simulink library "tpm"  (R2021b)
settings: Solver=VariableStepAuto  StartTime=0.0  StopTime=10.0  RelTol=1e-3
undefined symbols (not defined in the file or in its folder): ENUM_AN_LF, ENUM_AN_LR, ENUM_AN_RF, ENUM_AN_RR, ENUM_POWERSTA_OFF, ENUM_POWERSTA_OFFA, ENUM_POWERSTA_OFFC, ENUM_POWERSTA_ON, ENUM_POWERSTA_READY, ENUM_POWERSTA_STANDBY, ENUM_PWRSTASW_OFF, ENUM_PWRSTASW_OFFA, ENUM_PWRSTASW_OFFCHVCHRG, ENUM_PWRSTASW_STANDBY, ENUM_TPMSSNESORIDREGSTA_START, FALSE, KTPM_DataInVehSpdThreshold_kph, KTPM_Delay_raw8, KTPM_DiagLearn_flg, KTPM_TPMSModelVersion_raw, KTPM_TPMSModelVersionInit_raw, KTPM_WhlRotDir_enum_ovrdflg, KTPM_WhlRotDir_enum_ovrdval, TRUE, ZERO_FLOAT, ZERO_INT
libraries: simulink x58, $bdroot x27, hcu_lib x24
(part 8 of 9)

== stateflow chart tpm/TPM/TPMS/TPMS/Learn/AutoLocation/IDIdentify/Subsystem1/Chart ==
  state Sample [parallel]
    settings: executionOrder=1
    state DataNotEnough
    state Regisiter
      en:
      C=C+1;
      LFM=LF_PC;
      RFM=RF_PC;
      LRM=LR_PC;
      RRM=RR_PC;
    (default) -> DataNotEnough : {C=0;}
    Regisiter -> (junction 513) [order 2] : [GS]
    DataNotEnough -> Regisiter [order 2] : [!VINP_TPMSResButt_flg&&GS]
    (junction 513) -> (junction 514)
    (junction 514) -> Regisiter
    Regisiter -> DataNotEnough [order 1] : [VINP_TPMSResButt_flg]{C=0;}
    Regisiter -> (junction 528) [order 3] : [VPMM_PowerSta_enum!=ENUM_POWERSTA_ON&&...
        | VPMM_PowerSta_enum!=ENUM_POWERSTA_READY
        | ]
    (junction 528) -> (junction 532) : {C=0;}
    (junction 532) -> DataNotEnough
    DataNotEnough -> DataNotEnough [order 1] : [VINP_TPMSResButt_flg]{C=0;}
  data: VINP_TPMSResButt_flg input; VPMM_PowerSta_enum input; GS input; LR_PC input; LF_PC input; RR_PC input; RF_PC input; LFM output int16; LRM output int16; RRM output int16; RFM output int16; C output uint8; ENUM_POWERSTA_READY parameter; ENUM_POWERSTA_ON parameter

== matlab function tpm/TPM/TPMS/TPMS/Learn/AutoLocation/IDIdentify/Subsystem2/Enabled Subsystem1/MATLAB Function ==
  data: C input; S output; Min input; X2 input; X3 input; X4 input; Y2 output; Y3 output; Y4 output; X5 input; X6 input; X7 input; X8 input; X9 input; Y5 output; Y6 output; Y7 output; Y8 output; Y9 output
function [S,Y2,Y3,Y4,Y5,Y6,Y7,Y8,Y9]   = fcn(C,Min,X2,X3,X4,X5,X6,X7,X8,X9)
Y=int16([X2 X3 X4 X5 X6 X7 X8 X9 Min]);
if (C<9)
    S=300;
else
    B=sort(Y);
    D=zeros(1,length(B));
    for i=1:1:length(D)
        if (i~=length(D))
            D(i)=B(i+1)-B(i);
        else
            if (B(length(D))-B(1)>B(1)+96-B(length(D)))
                D(length(D))=B(1)+96-B(length(D));
            else
                D(length(D))=B(length(D))-B(1);
            end
        end
    end

    [K,I]=sort(D);
    S=sum(K(1:7));
end
Y2=Y(2);
Y3=Y(3);
Y4=Y(4);
Y5=Y(5);
Y6=Y(6);
Y7=Y(7);
Y8=Y(8);
Y9=Y(9);

== matlab function tpm/TPM/TPMS/TPMS/Learn/AutoLocation/IDIdentify/Subsystem2/Enabled Subsystem2/MATLAB Function ==
  data: C input; S output; Min input; X2 input; X3 input; X4 input; Y2 output; Y3 output; Y4 output; X5 input; X6 input; X7 input; X8 input; X9 input; Y5 output; Y6 output; Y7 output; Y8 output; Y9 output
function [S,Y2,Y3,Y4,Y5,Y6,Y7,Y8,Y9]   = fcn(C,Min,X2,X3,X4,X5,X6,X7,X8,X9)
Y=int16([X2 X3 X4 X5 X6 X7 X8 X9 Min]);
if (C<9)
    S=300;
else
    B=sort(Y);
    D=zeros(1,length(B));
    for i=1:1:length(D)
        if (i~=length(D))
            D(i)=B(i+1)-B(i);
        else
            if (B(length(D))-B(1)>B(1)+96-B(length(D)))
                D(length(D))=B(1)+96-B(length(D));
            else
                D(length(D))=B(length(D))-B(1);
            end
        end
    end

    [K,I]=sort(D);
    S=sum(K(1:7));
end
Y2=Y(2);
Y3=Y(3);
Y4=Y(4);
Y5=Y(5);
Y6=Y(6);
Y7=Y(7);
Y8=Y(8);
Y9=Y(9);

== matlab function tpm/TPM/TPMS/TPMS/Learn/AutoLocation/IDIdentify/Subsystem2/Enabled Subsystem3/MATLAB Function ==
  data: C input; S output; Min input; X2 input; X3 input; X4 input; Y2 output; Y3 output; Y4 output; X5 input; X6 input; X7 input; X8 input; X9 input; Y5 output; Y6 output; Y7 output; Y8 output; Y9 output
function [S,Y2,Y3,Y4,Y5,Y6,Y7,Y8,Y9]   = fcn(C,Min,X2,X3,X4,X5,X6,X7,X8,X9)
Y=int16([X2 X3 X4 X5 X6 X7 X8 X9 Min]);
if (C<9)
    S=300;
else
    B=sort(Y);
    D=zeros(1,length(B));
    for i=1:1:length(D)
        if (i~=length(D))
            D(i)=B(i+1)-B(i);
        else
            if (B(length(D))-B(1)>B(1)+96-B(length(D)))
                D(length(D))=B(1)+96-B(length(D));
            else
                D(length(D))=B(length(D))-B(1);
            end
        end
    end

    [K,I]=sort(D);
    S=sum(K(1:7));
end
Y2=Y(2);
Y3=Y(3);
Y4=Y(4);
Y5=Y(5);
Y6=Y(6);
Y7=Y(7);
Y8=Y(8);
Y9=Y(9);

== stateflow chart tpm/TPM/TPMS/TPMS/Learn/AutoLocation/Subsystem/Chart ==
  state writeSXID
    (default) -> (junction 6)
    writeSXID -> (junction 6)
    (junction 6) -> (junction 8) [order 1] : [VINP_TPMSResButt_flg]
    (junction 6) -> (junction 10) [order 2] : {
        | VTPM_FlashS1ID_raw=S1ID;
        | VTPM_FlashS2ID_raw=S2ID;
        | VTPM_FlashS3ID_raw=S3ID;
        | VTPM_FlashS4ID_raw=S4ID;
        | VTPM_FlashIDvalid_enum=1;
        | }
    (junction 8) -> (junction 12) : {
        | VTPM_FlashS1ID_raw=0;
        | VTPM_FlashS2ID_raw=0;
        | VTPM_FlashS3ID_raw=0;
        | VTPM_FlashS4ID_raw=0;
        | VTPM_FlashIDvalid_enum=0;
        | }
    (junction 12) -> (junction 10)
  data: S1ID input; S2ID input; S3ID input; S4ID input; VINP_TPMSResButt_flg input; VTPM_FlashS1ID_raw output uint32; VTPM_FlashS2ID_raw output uint32; VTPM_FlashS3ID_raw output uint32; VTPM_FlashS4ID_raw output uint32; VTPM_FlashIDvalid_enum output uint8

== matlab function tpm/TPM/TPMS/TPMS/Learn/AutoLocation/IDIdentify/Subsystem2/Enabled Subsystem5/MATLAB Function ==
  data: C input; S output; Min input; X2 input; X3 input; X4 input; Y2 output; Y3 output; Y4 output; X5 input; X6 input; X7 input; X8 input; X9 input; Y5 output; Y6 output; Y7 output; Y8 output; Y9 output
function [S,Y2,Y3,Y4,Y5,Y6,Y7,Y8,Y9]   = fcn(C,Min,X2,X3,X4,X5,X6,X7,X8,X9)
Y=int16([X2 X3 X4 X5 X6 X7 X8 X9 Min]);
if (C<9)
    S=300;
else
    B=sort(Y);
    D=zeros(1,length(B));
    for i=1:1:length(D)
        if (i~=length(D))
            D(i)=B(i+1)-B(i);
        else
            if (B(length(D))-B(1)>B(1)+96-B(length(D)))
                D(length(D))=B(1)+96-B(length(D));
            else
                D(length(D))=B(length(D))-B(1);
            end
        end
    end

    [K,I]=sort(D);
    S=sum(K(1:7));
end
Y2=Y(2);
Y3=Y(3);
Y4=Y(4);
Y5=Y(5);
Y6=Y(6);
Y7=Y(7);
Y8=Y(8);
Y9=Y(9);

== stateflow chart tpm/TPM/TPMS/TPMS/Learn/AutoLocation/IDIdentify/Subsystem3/Chart ==
  state Sample [parallel]
    settings: executionOrder=1
    state DataNotEnough
    state Regisiter
      en:
      C=C+1;
      LFM=LF_PC;
      RFM=RF_PC;
      LRM=LR_PC;
      RRM=RR_PC;
    (default) -> DataNotEnough : {C=0;}
    Regisiter -> (junction 513) [order 2] : [GS]
    DataNotEnough -> Regisiter [order 2] : [!VINP_TPMSResButt_flg&&GS]
    (junction 513) -> (junction 514)
    (junction 514) -> Regisiter
    Regisiter -> DataNotEnough [order 1] : [VINP_TPMSResButt_flg]{C=0;}
    Regisiter -> (junction 528) [order 3] : [VPMM_PowerSta_enum!=ENUM_POWERSTA_ON&&...
        | VPMM_PowerSta_enum!=ENUM_POWERSTA_READY
        | ]
    (junction 528) -> (junction 532) : {C=0;}
    (junction 532) -> DataNotEnough
    DataNotEnough -> DataNotEnough [order 1] : [VINP_TPMSResButt_flg]{C=0;}
  data: VINP_TPMSResButt_flg input; VPMM_PowerSta_enum input; GS input; LR_PC input; LF_PC input; RR_PC input; RF_PC input; LFM output int16; LRM output int16; RRM output int16; RFM output int16; C output uint8; ENUM_POWERSTA_READY parameter; ENUM_POWERSTA_ON parameter

== stateflow chart tpm/TPM/TPMS/TPMS/Learn/AutoLocation/IDIdentify/Subsystem3/Chart1 ==
  state GCal [parallel]
    settings: executionOrder=1
    state NoSignal
      en:G=false;
    state SignalIn
      en:G=true;
    (default) -> NoSignal
    NoSignal -> (junction 17) : [VINP_DATAin_flg]
    (junction 17) -> SignalIn [order 1] : [!Used]
    (junction 17) -> (junction 19) [order 2]
    (junction 19) -> NoSignal [order 2]
    (junction 19) -> SignalIn [order 1] : [VINP_IDin_raw32==IDout]
    SignalIn -> NoSignal
  state timecounter [parallel]
    settings: executionOrder=3
    state standby
      en:
      VTPM_S4timeout_flg=0;
      VTPM_timeout_cnt=0;
    state counter
      during:
      VTPM_timeout_cnt=VTPM_timeout_cnt+1;
    state stopcounter
    state timeout
      en:
      VTPM_S4timeout_flg=1;
    (default) -> standby
    (junction 68) -> standby
    (junction 63) -> (junction 68)
    standby -> counter : [Used&&!VTPM_FlashIDlock_flg]
    counter -> standby [order 1] : [!Used||(VINP_DATAin_flg&&IDout==VINP_IDin_raw32)]
    stopcounter -> counter : [VINP_VehSpeed_kph>=KTPM_DataInVehSpdThreshold_kph]
    counter -> stopcounter [order 3] : [VINP_VehSpeed_kph<KTPM_DataInVehSpdThreshold_kph]
    counter -> timeout [order 2] : [VTPM_timeout_cnt>12000]
    timeout -> (junction 63)
  state IDCheck [parallel]
    settings: executionOrder=2
    state FlashID
      en:
      IDout=VINP_S4ID_raw;
      Used=true;
      VTPM_S4IDLock_flg=true;
    state Unused
      en:IDout=0;
      VTPM_S4IDLock_flg=false;
      Used=false;
      IDLock_cnt=0;
    state VINP_DATAin_flg
      state Used
        en:IDout=VINP_IDin_raw32;
        Used=true;
        IDLock_cnt=IDLock_cnt+1;
      state Lock
        en:VTPM_S4IDLock_flg=true;
      Used -> Used [order 2] : [VINP_DATAin_flg&&IDout==VINP_IDin_raw32]
      Used -> Lock [order 1] : [IDLock_cnt>=4]
    (default) -> Unused
    Unused -> FlashID [order 1] : [VTPM_FlashIDlock_flg||VTPM_TPMSmanualDone_flg]
    FlashID -> Unused : [VINP_TPMSResButt_flg]
    Unused -> Used [order 2] : [VINP_DATAin_flg]
    Used -> Unused [order 3] : [VTPM_S4timeout_flg==1]
    VINP_DATAin_flg -> FlashID [order 2] : [VTPM_TPMSmanualDone_flg]
    VINP_DATAin_flg -> Unused [order 1] : [VINP_TPMSResButt_flg]
  data: VINP_IDin_raw32 input; VINP_TPMSResButt_flg input; VINP_DATAin_flg input; G output boolean; Used output boolean; VTPM_S4IDLock_flg output boolean; IDout output uint32; VTPM_FlashIDlock_flg input; VINP_S4ID_raw input; VINP_VehSpeed_kph input; IDLock_cnt local double; VTPM_timeout_cnt local double; VTPM_S4timeout_flg output boolean; VTPM_TPMSmanualDone_flg input; KTPM_DataInVehSpdThreshold_kph input

== matlab function tpm/TPM/TPMS/TPMS/Learn/AutoLocation/IDIdentify/Subsystem3/Enabled Subsystem1/MATLAB Function ==
  data: C input; S output; Min input; X2 input; X3 input; X4 input; Y2 output; Y3 output; Y4 output; X5 input; X6 input; X7 input; X8 input; X9 input; Y5 output; Y6 output; Y7 output; Y8 output; Y9 output
function [S,Y2,Y3,Y4,Y5,Y6,Y7,Y8,Y9]   = fcn(C,Min,X2,X3,X4,X5,X6,X7,X8,X9)
Y=int16([X2 X3 X4 X5 X6 X7 X8 X9 Min]);
if (C<9)
    S=300;
else
    B=sort(Y);
    D=zeros(1,length(B));
    for i=1:1:length(D)
        if (i~=length(D))
            D(i)=B(i+1)-B(i);
        else
            if (B(length(D))-B(1)>B(1)+96-B(length(D)))
                D(length(D))=B(1)+96-B(length(D));
            else
                D(length(D))=B(length(D))-B(1);
            end
        end
    end

    [K,I]=sort(D);
    S=sum(K(1:7));
end
Y2=Y(2);
Y3=Y(3);
Y4=Y(4);
Y5=Y(5);
Y6=Y(6);
Y7=Y(7);
Y8=Y(8);
Y9=Y(9);

== matlab function tpm/TPM/TPMS/TPMS/Learn/AutoLocation/IDIdentify/Subsystem3/Enabled Subsystem2/MATLAB Function ==
  data: C input; S output; Min input; X2 input; X3 input; X4 input; Y2 output; Y3 output; Y4 output; X5 input; X6 input; X7 input; X8 input; X9 input; Y5 output; Y6 output; Y7 output; Y8 output; Y9 output
function [S,Y2,Y3,Y4,Y5,Y6,Y7,Y8,Y9]   = fcn(C,Min,X2,X3,X4,X5,X6,X7,X8,X9)
Y=int16([X2 X3 X4 X5 X6 X7 X8 X9 Min]);
if (C<9)
    S=300;
else
    B=sort(Y);
    D=zeros(1,length(B));
    for i=1:1:length(D)
        if (i~=length(D))
            D(i)=B(i+1)-B(i);
        else
            if (B(length(D))-B(1)>B(1)+96-B(length(D)))
                D(length(D))=B(1)+96-B(length(D));
            else
                D(length(D))=B(length(D))-B(1);
            end
        end
    end

    [K,I]=sort(D);
    S=sum(K(1:7));
end
Y2=Y(2);
Y3=Y(3);
Y4=Y(4);
Y5=Y(5);
Y6=Y(6);
Y7=Y(7);
Y8=Y(8);
Y9=Y(9);

== matlab function tpm/TPM/TPMS/TPMS/Learn/AutoLocation/IDIdentify/Subsystem3/Enabled Subsystem3/MATLAB Function ==
  data: C input; S output; Min input; X2 input; X3 input; X4 input; Y2 output; Y3 output; Y4 output; X5 input; X6 input; X7 input; X8 input; X9 input; Y5 output; Y6 output; Y7 output; Y8 output; Y9 output
function [S,Y2,Y3,Y4,Y5,Y6,Y7,Y8,Y9]   = fcn(C,Min,X2,X3,X4,X5,X6,X7,X8,X9)
Y=int16([X2 X3 X4 X5 X6 X7 X8 X9 Min]);
if (C<9)
    S=300;
else
    B=sort(Y);
    D=zeros(1,length(B));
    for i=1:1:length(D)
        if (i~=length(D))
            D(i)=B(i+1)-B(i);
        else
            if (B(length(D))-B(1)>B(1)+96-B(length(D)))
                D(length(D))=B(1)+96-B(length(D));
            else
                D(length(D))=B(length(D))-B(1);
            end
        end
    end

    [K,I]=sort(D);
    S=sum(K(1:7));
end
Y2=Y(2);
Y3=Y(3);
Y4=Y(4);
Y5=Y(5);
Y6=Y(6);
Y7=Y(7);
Y8=Y(8);
Y9=Y(9);

== stateflow chart tpm/TPM/TPMS/TPMS/Learn/AutoLocation/IDIdentify/Subsystem7/Chart1 ==
  state GCal [parallel]
    settings: executionOrder=1
    state NoSignal
      en:G=false;
    state SignalIn
      en:G=true;
    (default) -> NoSignal
    NoSignal -> (junction 17) : [VINP_DATAin_flg]
    (junction 17) -> SignalIn [order 1] : [!Used]
    (junction 17) -> (junction 19) [order 2]
    (junction 19) -> NoSignal [order 2]
    (junction 19) -> SignalIn [order 1] : [VINP_IDin_raw32==IDout]
    SignalIn -> NoSignal
  state timecounter [parallel]
    settings: executionOrder=3
    state standby
      en:
      VTPM_S1timeout_flg=0;
      VTPM_timeout_cnt=0;
    state counter
      during:
      VTPM_timeout_cnt=VTPM_timeout_cnt+1;
    state stopcounter
    state timeout
      en:
      VTPM_S1timeout_flg=1;
    (default) -> standby
    (junction 65) -> standby
    (junction 60) -> (junction 65)
    standby -> counter : [Used&&!VTPM_FlashIDlock_flg]
    counter -> standby [order 1] : [!Used||(VINP_DATAin_flg&&IDout==VINP_IDin_raw32)]
    stopcounter -> counter : [VINP_VehSpeed_kph>=KTPM_DataInVehSpdThreshold_kph]
    counter -> stopcounter [order 3] : [VINP_VehSpeed_kph<KTPM_DataInVehSpdThreshold_kph]
    counter -> timeout [order 2] : [VTPM_timeout_cnt>12000]
    timeout -> (junction 60)
  state IDCheck [parallel]
    settings: executionOrder=2
    state Unused
      en:IDout=0;
      VTPM_S1IDLock_flg=false;
      Used=false;
      VTPM_IDLock_cnt=0;
    state FlashID
      en:
      IDout=VINP_S1ID_raw;
      Used=true;
      VTPM_S1IDLock_flg=true;
    state VINP_DATAin_flg
      state Used
        en:IDout=VINP_IDin_raw32;
        Used=true;
        VTPM_IDLock_cnt+=1;
      state Lock
        en:VTPM_S1IDLock_flg=true;
      Used -> Used [order 2] : [VINP_DATAin_flg&&IDout==VINP_IDin_raw32]
      Used -> Lock [order 1] : [VTPM_IDLock_cnt>=4]
    (default) -> Unused
    Unused -> FlashID [order 1] : [VTPM_FlashIDlock_flg||VTPM_TPMSmanualDone_flg]
    FlashID -> Unused : [VINP_TPMSResButt_flg]
    Unused -> Used [order 2] : [VINP_DATAin_flg]
    Used -> Unused [order 3] : [VTPM_S1timeout_flg==1]
    VINP_DATAin_flg -> FlashID [order 2] : [VTPM_TPMSmanualDone_flg]
    VINP_DATAin_flg -> Unused [order 1] : [VINP_TPMSResButt_flg]
  data: VINP_IDin_raw32 input; VINP_TPMSResButt_flg input; VINP_DATAin_flg input; G output boolean; Used output boolean; VTPM_S1IDLock_flg output boolean; IDout output uint32; VTPM_FlashIDlock_flg input; VINP_S1ID_raw input; VINP_VehSpeed_kph input; VTPM_IDLock_cnt local uint32; VTPM_timeout_cnt local uint32; VTPM_S1timeout_flg output boolean; VTPM_TPMSmanualDone_flg input; KTPM_DataInVehSpdThreshold_kph input

== stateflow chart tpm/TPM/TPMS/TPMS/Learn/AutoLocation/Doublecheck/Chart ==
  (default) -> (junction 18)
  (junction 18) -> (junction 19) [order 1] : [VTPM_SaveToRAM_flg]
  (junction 18) -> (junction 36) [order 2]
  (junction 19) -> (junction 23) : {
      |  VTPM_ChkLFID_raw=VTPM_LFID_raw;
      |  VTPM_ChkRFID_raw=VTPM_RFID_raw;
      |  VTPM_ChkLRID_raw=VTPM_LRID_raw;
      |  VTPM_ChkRRID_raw=VTPM_RRID_raw;
      | }
  (junction 23) -> (junction 36)
  data: VTPM_LFID_raw input; VTPM_RFID_raw input; VTPM_LRID_raw input; VTPM_RRID_raw input; VTPM_ChkLFID_raw output uint32; VTPM_ChkRFID_raw output uint32; VTPM_ChkLRID_raw output uint32; VTPM_ChkRRID_raw output uint32; VTPM_SaveToRAM_flg input

== stateflow chart tpm/TPM/TPMS/TPMS/Learn/AutoLocation/IDIdentify/Subsystem1/Chart1 ==
  state GCal [parallel]
    settings: executionOrder=1
    state NoSignal
      en:G=false;
    state SignalIn
      en:G=true;
    (default) -> NoSignal
    NoSignal -> (junction 17) : [VINP_DATAin_flg]
    (junction 17) -> SignalIn [order 1] : [!Used]
    (junction 17) -> (junction 19) [order 2]
    (junction 19) -> NoSignal [order 2]
    (junction 19) -> SignalIn [order 1] : [VINP_IDin_raw32==IDout]
    SignalIn -> NoSignal
  state IDCheck [parallel]
    settings: executionOrder=2
    state Unused
      en:IDout=0;
      VTPM_S2IDLock_flg=false;
      Used=false;
      IDLock_cnt=0;
    state FlashID
      en:
      IDout=VINP_S2ID_raw;
      Used=true;
      VTPM_S2IDLock_flg=true;
    state VINP_DATAin_flg
      state Used
        en:IDout=VINP_IDin_raw32;
        Used=true;
        IDLock_cnt+=1;
      state Lock
        en:VTPM_S2IDLock_flg=true;
      Used -> Used [order 2] : [VINP_DATAin_flg&&IDout==VINP_IDin_raw32]
      Used -> Lock [order 1] : [IDLock_cnt>=4]
    (default) -> Unused
    Unused -> FlashID [order 1] : [VTPM_FlashIDlock_flg||VTPM_TPMSmanualDone_flg]
    FlashID -> Unused : [VINP_TPMSResButt_flg]
    VINP_DATAin_flg -> FlashID [order 2] : [VTPM_TPMSmanualDone_flg]
    Unused -> Used [order 2] : [VINP_DATAin_flg]
    Used -> Unused [order 3] : [VTPM_S2timeout_flg==1]
    VINP_DATAin_flg -> Unused [order 1] : [VINP_TPMSResButt_flg]
  state timecounter [parallel]
    settings: executionOrder=3
    state standby
      en:
      VTPM_S2timeout_flg=0;
      VTPM_timeout_cnt=0;
    state counter
      during:
      VTPM_timeout_cnt=VTPM_timeout_cnt+1;
    state stopcounter
    state timeout
      en:
      VTPM_S2timeout_flg=1;
    (default) -> standby
    (junction 76) -> standby
    (junction 74) -> (junction 76)
    standby -> counter : [Used&&!VTPM_FlashIDlock_flg]
    counter -> standby [order 1] : [!Used||(VINP_DATAin_flg&&IDout==VINP_IDin_raw32)]
    stopcounter -> counter : [VINP_VehSpeed_kph>=KTPM_DataInVehSpdThreshold_kph]
    counter -> stopcounter [order 3] : [VINP_VehSpeed_kph<KTPM_DataInVehSpdThreshold_kph]
    counter -> timeout [order 2] : [VTPM_timeout_cnt>12000]
    timeout -> (junction 74)
  data: VINP_IDin_raw32 input; VINP_TPMSResButt_flg input; VINP_DATAin_flg input; G output boolean; Used output boolean; VTPM_S2IDLock_flg output boolean; IDout output uint32; VTPM_FlashIDlock_flg input; VINP_S2ID_raw input; VINP_VehSpeed_kph input; IDLock_cnt local uint32; VTPM_timeout_cnt local uint32; VTPM_S2timeout_flg output boolean; VTPM_TPMSmanualDone_flg input; KTPM_DataInVehSpdThreshold_kph input single

== matlab function tpm/TPM/TPMS/TPMS/Learn/AutoLocation/IDIdentify/Subsystem1/Enabled Subsystem1/MATLAB Function ==
  data: C input; S output; Min input; X2 input; X3 input; X4 input; Y2 output; Y3 output; Y4 output; X5 input; X6 input; X7 input; X8 input; X9 input; Y5 output; Y6 output; Y7 output; Y8 output; Y9 output
function [S,Y2,Y3,Y4,Y5,Y6,Y7,Y8,Y9]   = fcn(C,Min,X2,X3,X4,X5,X6,X7,X8,X9)
Y=int16([X2 X3 X4 X5 X6 X7 X8 X9 Min]);
if (C<9)
    S=300;
else
    B=sort(Y);
    D=zeros(1,length(B));
    for i=1:1:length(D)
        if (i~=length(D))
            D(i)=B(i+1)-B(i);
        else
            if (B(length(D))-B(1)>B(1)+96-B(length(D)))
                D(length(D))=B(1)+96-B(length(D));
            else
                D(length(D))=B(length(D))-B(1);
            end
        end
    end

    [K,I]=sort(D);
    S=sum(K(1:7));
end
Y2=Y(2);
Y3=Y(3);
Y4=Y(4);
Y5=Y(5);
Y6=Y(6);
Y7=Y(7);
Y8=Y(8);
Y9=Y(9);

== matlab function tpm/TPM/TPMS/TPMS/Learn/AutoLocation/IDIdentify/Subsystem1/Enabled Subsystem2/MATLAB Function ==
  data: C input; S output; Min input; X2 input; X3 input; X4 input; Y2 output; Y3 output; Y4 output; X5 input; X6 input; X7 input; X8 input; X9 input; Y5 output; Y6 output; Y7 output; Y8 output; Y9 output
function [S,Y2,Y3,Y4,Y5,Y6,Y7,Y8,Y9]   = fcn(C,Min,X2,X3,X4,X5,X6,X7,X8,X9)
Y=int16([X2 X3 X4 X5 X6 X7 X8 X9 Min]);
if (C<9)
    S=300;
else
    B=sort(Y);
    D=zeros(1,length(B));
    for i=1:1:length(D)
        if (i~=length(D))
            D(i)=B(i+1)-B(i);
        else
            if (B(length(D))-B(1)>B(1)+96-B(length(D)))
                D(length(D))=B(1)+96-B(length(D));
            else
                D(length(D))=B(length(D))-B(1);
            end
        end
    end

    [K,I]=sort(D);
    S=sum(K(1:7));
end
Y2=Y(2);
Y3=Y(3);
Y4=Y(4);
Y5=Y(5);
Y6=Y(6);
Y7=Y(7);
Y8=Y(8);
Y9=Y(9);

== matlab function tpm/TPM/TPMS/TPMS/Learn/AutoLocation/IDIdentify/Subsystem1/Enabled Subsystem3/MATLAB Function ==
  data: C input; S output; Min input; X2 input; X3 input; X4 input; Y2 output; Y3 output; Y4 output; X5 input; X6 input; X7 input; X8 input; X9 input; Y5 output; Y6 output; Y7 output; Y8 output; Y9 output
function [S,Y2,Y3,Y4,Y5,Y6,Y7,Y8,Y9]   = fcn(C,Min,X2,X3,X4,X5,X6,X7,X8,X9)
Y=int16([X2 X3 X4 X5 X6 X7 X8 X9 Min]);
if (C<9)
    S=300;
else
    B=sort(Y);
    D=zeros(1,length(B));
    for i=1:1:length(D)
        if (i~=length(D))
            D(i)=B(i+1)-B(i);
        else
            if (B(length(D))-B(1)>B(1)+96-B(length(D)))
                D(length(D))=B(1)+96-B(length(D));
            else
                D(length(D))=B(length(D))-B(1);
            end
        end
    end

    [K,I]=sort(D);
    S=sum(K(1:7));
end
Y2=Y(2);
Y3=Y(3);
Y4=Y(4);
Y5=Y(5);
Y6=Y(6);
Y7=Y(7);
Y8=Y(8);
Y9=Y(9);

== matlab function tpm/TPM/TPMS/TPMS/Learn/AutoLocation/IDIdentify/Subsystem1/Enabled Subsystem5/MATLAB Function ==
  data: C input; S output; Min input; X2 input; X3 input; X4 input; Y2 output; Y3 output; Y4 output; X5 input; X6 input; X7 input; X8 input; X9 input; Y5 output; Y6 output; Y7 output; Y8 output; Y9 output
function [S,Y2,Y3,Y4,Y5,Y6,Y7,Y8,Y9]   = fcn(C,Min,X2,X3,X4,X5,X6,X7,X8,X9)
Y=int16([X2 X3 X4 X5 X6 X7 X8 X9 Min]);
if (C<9)
    S=300;
else
    B=sort(Y);
    D=zeros(1,length(B));
    for i=1:1:length(D)
        if (i~=length(D))
            D(i)=B(i+1)-B(i);
        else
            if (B(length(D))-B(1)>B(1)+96-B(length(D)))
                D(length(D))=B(1)+96-B(length(D));
            else
                D(length(D))=B(length(D))-B(1);
            end
        end
    end

    [K,I]=sort(D);
    S=sum(K(1:7));
end
Y2=Y(2);
Y3=Y(3);
Y4=Y(4);
Y5=Y(5);
Y6=Y(6);
Y7=Y(7);
Y8=Y(8);
Y9=Y(9);

== stateflow chart tpm/TPM/TPMS/TPMS/Send/DATA/Chart ==
  state read
    (default) -> (junction 7) : {
        | VTPM_PreS1Pressure_raw=VINP_FlashLFWheelPress_raw8;
        | VTPM_PreS2Pressure_raw=VINP_FlashRFWheelPress_raw8;
        | VTPM_PreS3Pressure_raw=VINP_FlashLRWheelPress_raw8;
        | VTPM_PreS4Pressure_raw=VINP_FlashRRWheelPress_raw8;
        | VTPM_PreS1Temp_raw=VINP_FlashLFWheelTemp_C;
        | VTPM_PreS2Temp_raw=VINP_FlashRFWheelTemp_C;
        | VTPM_PreS3Temp_raw=VINP_FlashLRWheelTemp_C;
        | VTPM_PreS4Temp_raw=VINP_FlashRRWheelTemp_C;
        | }
    read -> (junction 7) [order 2] : [VINP_DATAin_flg||VINP_TPMSResButt_flg]
    (junction 7) -> (junction 9) [order 1] : [VINP_IDin_raw32==VTPM_S1ID_raw32&&VTPM_IDLOCK_flg&&VINP_DATAin_flg]
    (junction 7) -> (junction 11) [order 2]
    (junction 9) -> (junction 27) : {VTPM_PreS1Pressure_raw=VINP_Pin_raw8;
        |  VTPM_PreS1Temp_raw=VINP_Tin_raw8;
        |  VTPM_PreS1readdone_flg=true;
        | }
    (junction 11) -> (junction 13) [order 1] : [VINP_IDin_raw32==VTPM_S2ID_raw32&&VTPM_IDLOCK_flg&&VINP_DATAin_flg]
    (junction 11) -> (junction 15) [order 2]
    (junction 13) -> (junction 30) : {VTPM_PreS2Pressure_raw=VINP_Pin_raw8;
        |  VTPM_PreS2Temp_raw=VINP_Tin_raw8;
        |  VTPM_PreS2readdone_flg=true;
        | }
    (junction 15) -> (junction 17) [order 1] : [VINP_IDin_raw32==VTPM_S3ID_raw32&&VTPM_IDLOCK_flg&&VINP_DATAin_flg]
    (junction 15) -> (junction 19) [order 2]
    (junction 17) -> (junction 32) : {VTPM_PreS3Pressure_raw=VINP_Pin_raw8;
        |  VTPM_PreS3Temp_raw=VINP_Tin_raw8;
        |  VTPM_PreS3readdone_flg=true;
        | }
    (junction 19) -> (junction 21) [order 1] : [VINP_IDin_raw32==VTPM_S4ID_raw32&&VTPM_IDLOCK_flg&&VINP_DATAin_flg]
    (junction 19) -> (junction 25) [order 2]
    (junction 21) -> (junction 34) : {VTPM_PreS4Pressure_raw=VINP_Pin_raw8;
        |  VTPM_PreS4Temp_raw=VINP_Tin_raw8;
        |  VTPM_PreS4readdone_flg=true;
        | }
    (junction 34) -> (junction 25)
    (junction 32) -> (junction 34)
    (junction 30) -> (junction 32)
    (junction 27) -> (junction 30)
    (junction 25) -> (junction 102)
    read -> (junction 102) [order 1] : [VTPM_TPMSmanualDone_flg]
    (junction 102) -> (junction 109) [order 1] : [VTPM_TPMSmanualDone_flg]
    (junction 102) -> (junction 82) [order 2]
    (junction 109) -> (junction 111) : {VTPM_PreS1Pressure_raw=VTPM_ManualID1pressure_raw;
        |  VTPM_PreS2Pressure_raw=VTPM_ManualID2pressure_raw;
        |  VTPM_PreS3Pressure_raw=VTPM_ManualID3pressure_raw;
        |  VTPM_PreS4Pressure_raw=VTPM_ManualID4pressure_raw;
        |  VTPM_PreS1Temp_raw=VTPM_ManualID1Temp_C;
        |  VTPM_PreS2Temp_raw=VTPM_ManualID2Temp_C;
        |  VTPM_PreS3Temp_raw=VTPM_ManualID3Temp_C;
        |  VTPM_PreS4Temp_raw=VTPM_ManualID4Temp_C;
        |  VTPM_PreS1readdone_flg=true;
        |  VTPM_PreS2readdone_flg=true;
        |  VTPM_PreS3readdone_flg=true;
        |  VTPM_PreS4readdone_flg=true;
        | }
    (junction 82) -> (junction 84) [order 1] : [VINP_TPMSResButt_flg]
    (junction 82) -> (junction 88) [order 2]
    (junction 84) -> (junction 86) : {
        | VTPM_PreS1Pressure_raw=0;
        | VTPM_PreS2Pressure_raw=0;
        | VTPM_PreS3Pressure_raw=0;
        | VTPM_PreS4Pressure_raw=0;
        | VTPM_PreS1Temp_raw=215;
        | VTPM_PreS2Temp_raw=215;
        | VTPM_PreS3Temp_raw=215;
        | VTPM_PreS4Temp_raw=215;
        | VTPM_PreS1readdone_flg=false;
        | VTPM_PreS2readdone_flg=false;
        | VTPM_PreS3readdone_flg=false;
        | VTPM_PreS4readdone_flg=false;
        | }
  data: VINP_DATAin_flg input; VTPM_S1ID_raw32 input; VTPM_S2ID_raw32 input; VTPM_S3ID_raw32 input; VTPM_S4ID_raw32 input; VINP_IDin_raw32 input; VTPM_IDLOCK_flg input; VINP_Pin_raw8 input; VTPM_PreS1Pressure_raw output uint8; VTPM_PreS2Pressure_raw output uint8; VTPM_PreS4Pressure_raw output uint8; VTPM_PreS3Pressure_raw output uint8; VINP_Tin_raw8 input; VTPM_PreS1Temp_raw output single; VTPM_PreS2Temp_raw output single; VTPM_PreS3Temp_raw output single; VTPM_PreS4Temp_raw output single; VTPM_PreS1readdone_flg output boolean; VTPM_PreS2readdone_flg output boolean; VTPM_PreS3readdone_flg output boolean; VINP_FlashLFWheelPress_raw8 input; VINP_FlashRFWheelPress_raw8 input; VINP_FlashLRWheelPress_raw8 input; VINP_FlashRRWheelPress_raw8 input; VINP_FlashLFWheelTemp_C input; VINP_FlashRFWheelTemp_C input; VINP_FlashLRWheelTemp_C input; VINP_FlashRRWheelTemp_C input; VINP_TPMSResButt_flg input; VTPM_PreS4readdone_flg output boolean; VTPM_ManualID1pressure_raw input; VTPM_ManualID2pressure_raw input; VTPM_ManualID3pressure_raw input; VTPM_ManualID4pressure_raw input; VTPM_ManualID1Temp_C input; VTPM_ManualID2Temp_C input; VTPM_ManualID3Temp_C input; VTPM_ManualID4Temp_C input; VTPM_TPMSmanualDone_flg input

== matlab function tpm/TPM/TPMS/TPMS/Learn/AutoLocation/IDIdentify/Subsystem3/Enabled Subsystem5/MATLAB Function ==
  data: C input; S output; Min input; X2 input; X3 input; X4 input; Y2 output; Y3 output; Y4 output; X5 input; X6 input; X7 input; X8 input; X9 input; Y5 output; Y6 output; Y7 output; Y8 output; Y9 output
function [S,Y2,Y3,Y4,Y5,Y6,Y7,Y8,Y9]   = fcn(C,Min,X2,X3,X4,X5,X6,X7,X8,X9)
Y=int16([X2 X3 X4 X5 X6 X7 X8 X9 Min]);
if (C<9)
    S=300;
else
    B=sort(Y);
    D=zeros(1,length(B));
    for i=1:1:length(D)
        if (i~=length(D))
            D(i)=B(i+1)-B(i);
        else
            if (B(length(D))-B(1)>B(1)+96-B(length(D)))
                D(length(D))=B(1)+96-B(length(D));
            else
                D(length(D))=B(length(D))-B(1);
            end
        end
    end

    [K,I]=sort(D);
    S=sum(K(1:7));
end
Y2=Y(2);
Y3=Y(3);
Y4=Y(4);
Y5=Y(5);
Y6=Y(6);
Y7=Y(7);
Y8=Y(8);
Y9=Y(9);

== stateflow chart tpm/TPM/TPMS/TPMS/Learn/AutoLocation/IDIdentify/Acceptancerate/Chart2 ==
  state SensorReceived [parallel]
    settings: executionOrder=1
    state VINP_TPMSResButt_flg
      en:
      COUNT1=0;
      ID1_message_ALTU=0;
      C=0;
      STOP=0;
      BackFlg=0;
    state NoSignal
    state VINP_FAT_flg1
      en:
      COUNT1=COUNT1 +1
      C=0
    state VINP_FAT_flg0
      en:
      C=C+1
      ID1_message_ALTU=ID1_message_ALTU+1
    state fivesec
    (default) -> VINP_TPMSResButt_flg
    VINP_TPMSResButt_flg -> NoSignal
    NoSignal -> VINP_TPMSResButt_flg [order 1] : [VINP_TPMSResButt_flg||BackFlg==1]
    NoSignal -> (junction 57) [order 2] : [VINP_DATAin_flg&VINP_IDin_raw32==IDout&S1IDLock&VINP_FAT_flg==1&STOP==0]
    NoSignal -> (junction 61) [order 3] : [VINP_DATAin_flg&VINP_IDin_raw32==IDout&S1IDLock&VINP_FAT_flg==0]
    (junction 57) -> VINP_FAT_flg1
    (junction 61) -> VINP_FAT_flg0
    (junction 97) -> NoSignal : {COUNT1=0,ID1_message_ALTU=0,C=0,STOP=0}
    fivesec -> NoSignal [order 2]
    fivesec -> NoSignal [order 1] : [C==5]{STOP=1;C=0;}
    (junction 105) -> NoSignal : {COUNT1=0,ID1_message_ALTU=0,C=0,STOP=0}
    VINP_FAT_flg1 -> (junction 97) [order 1] : [VINP_TPMSResButt_flg||COUNT1==40||BackFlg==1]
    VINP_FAT_flg0 -> (junction 105) [order 1] : [VINP_TPMSResButt_flg||BackFlg==1]
    VINP_FAT_flg1 -> fivesec [order 2] : [after(500,tick)]
    VINP_FAT_flg0 -> fivesec [order 2] : [after(500,tick)]
  state time_cal [parallel]
    settings: executionOrder=2
    state cal1
      en:
      time_cal=time_cal+1
    state default
      en:
      time_cal=0
      BackFlg=0
    state back
      en:
      BackFlg=1
    (default) -> default
    default -> cal1 : [after(6400,tick)]{BackFlg=0}
    back -> default
    cal1 -> back [order 1] : [VINP_TPMSResButt_flg||time_cal>9]
    cal1 -> cal1 [order 2] : [after(6400,tick)]
  data: VINP_IDin_raw32 input; VINP_TPMSResButt_flg input; VINP_DATAin_flg input; S1IDLock input; COUNT1 output uint8; VINP_FAT_flg input; IDout input; ID1_message_ALTU output uint8; STOP local boolean; C local uint8; time_cal local uint8; BackFlg local boolean

== stateflow chart tpm/TPM/TPMS/TPMS/Learn/AutoLocation/IDIdentify/Acceptancerate/Chart3 ==
  state SensorReceived [parallel]
    settings: executionOrder=1
    state VINP_TPMSResButt_flg
      en:
      COUNT2=0;
      ID2_message_ALTU=0;
      C=0;
      STOP=0;
      BackFlg=0;
    state NoSignal
    state VINP_FAT_flg1
      en:
      COUNT2=COUNT2 +1
      C=0
    state VINP_FAT_flg0
      en:
      C=C+1
      ID2_message_ALTU=ID2_message_ALTU+1
    state fivesec
    (default) -> VINP_TPMSResButt_flg
    VINP_TPMSResButt_flg -> NoSignal
    NoSignal -> VINP_TPMSResButt_flg [order 1] : [VINP_TPMSResButt_flg||BackFlg==1]
    NoSignal -> (junction 57) [order 2] : [VINP_DATAin_flg&VINP_IDin_raw32==IDout&S2IDLock&VINP_FAT_flg==1&STOP==0]
    NoSignal -> (junction 61) [order 3] : [VINP_DATAin_flg&VINP_IDin_raw32==IDout&S2IDLock&VINP_FAT_flg==0]
    (junction 57) -> VINP_FAT_flg1
    (junction 61) -> VINP_FAT_flg0
    (junction 97) -> NoSignal : {COUNT2=0,ID2_message_ALTU=0,C=0,STOP=0}
    fivesec -> NoSignal [order 2]
    fivesec -> NoSignal [order 1] : [C==5]{STOP=1;C=0;}
    (junction 105) -> NoSignal : {COUNT2=0,ID2_message_ALTU=0,C=0,STOP=0}
    VINP_FAT_flg1 -> (junction 97) [order 1] : [VINP_TPMSResButt_flg||COUNT2==40||BackFlg==1]
    VINP_FAT_flg0 -> (junction 105) [order 1] : [VINP_TPMSResButt_flg||BackFlg==1]
    VINP_FAT_flg1 -> fivesec [order 2] : [after(500,tick)]
    VINP_FAT_flg0 -> fivesec [order 2] : [after(500,tick)]
  state time_cal [parallel]
    settings: executionOrder=2
    state cal1
      en:
      time_cal=time_cal+1
    state default
      en:
      time_cal=0
      BackFlg=0
    state back
      en:
      BackFlg=1
    (default) -> default
    default -> cal1 : [after(6400,tick)]{BackFlg=0}
    back -> default
    cal1 -> back [order 1] : [VINP_TPMSResButt_flg||time_cal>9]
    cal1 -> cal1 [order 2] : [after(6400,tick)]
  data: VINP_IDin_raw32 input; VINP_TPMSResButt_flg input; VINP_DATAin_flg input; VINP_FAT_flg input; IDout input; STOP local boolean; C local uint8; ID2_message_ALTU output uint8; COUNT2 output uint8; S2IDLock input; BackFlg local boolean; time_cal local uint8

== stateflow chart tpm/TPM/TPMS/TPMS/Learn/AutoLocation/IDIdentify/IDLOCK ==
  state DataSwitch
    (default) -> (junction 5)
    DataSwitch -> (junction 42)
    (junction 42) -> (junction 5) [order 1] : [VINP_DATAin_flg]
    (junction 5) -> (junction 7) [order 1] : [used1&&VINP_IDin_raw32==IDout1]{DATAout=1;}
    (junction 42) -> (junction 44) [order 2] : {DATAout=0;}
    (junction 5) -> (junction 9) [order 2]
    (junction 9) -> (junction 11) [order 1] : [used2&&VINP_IDin_raw32==IDout2]{DATAout=2;}
    (junction 9) -> (junction 13) [order 2]
    (junction 13) -> (junction 15) [order 1] : [used3&&VINP_IDin_raw32==IDout3]{DATAout=3;}
    (junction 13) -> (junction 17) [order 2]
    (junction 17) -> (junction 19) [order 1] : [used4&&VINP_IDin_raw32==IDout4]{DATAout=4;}
    (junction 17) -> (junction 24) [order 2]
    (junction 24) -> (junction 26) [order 1] : [!used1]{DATAout=1;}
    (junction 24) -> (junction 28) [order 2]
    (junction 28) -> (junction 30) [order 1] : [!used2]{DATAout=2;}
    (junction 28) -> (junction 32) [order 2]
    (junction 32) -> (junction 34) [order 1] : [!used3]{DATAout=3;}
    (junction 32) -> (junction 36) [order 2]
    (junction 36) -> (junction 38) [order 1] : [!used4]{DATAout=4;}
    (junction 36) -> (junction 40) [order 2] : {DATAout=0;}
  data: VINP_DATAin_flg input; used1 input; used2 input; used3 input; used4 input; IDout1 input; IDout2 input; IDout3 input; IDout4 input; VINP_IDin_raw32 input; DATAout output uint8

== stateflow chart tpm/TPM/TPMS/TPMS/Learn/AutoLocation/IDIdentify/Acceptancerate/Chart4 ==
  state SensorReceived [parallel]
    settings: executionOrder=1
    state VINP_TPMSResButt_flg
      en:
      COUNT3=0;
      ID3_message_ALTU=0;
      C=0;
      STOP=0;
      BackFlg=0;
    state NoSignal
    state VINP_FAT_flg1
      en:
      COUNT3=COUNT3 +1
      C=0
    state VINP_FAT_flg0
      en:
      C=C+1
      ID3_message_ALTU=ID3_message_ALTU+1
    state fivesec
    (default) -> VINP_TPMSResButt_flg
    VINP_TPMSResButt_flg -> NoSignal
    NoSignal -> VINP_TPMSResButt_flg [order 1] : [VINP_TPMSResButt_flg||BackFlg==1]
    NoSignal -> (junction 57) [order 2] : [VINP_DATAin_flg&VINP_IDin_raw32==IDout&S3IDLock&VINP_FAT_flg==1&STOP==0]
    NoSignal -> (junction 61) [order 3] : [VINP_DATAin_flg&VINP_IDin_raw32==IDout&S3IDLock&VINP_FAT_flg==0]
    (junction 57) -> VINP_FAT_flg1
    (junction 61) -> VINP_FAT_flg0
    (junction 97) -> NoSignal : {COUNT3=0,ID3_message_ALTU=0,C=0,STOP=0}
    fivesec -> NoSignal [order 2]
    fivesec -> NoSignal [order 1] : [C==5]{STOP=1;C=0;}
    (junction 105) -> NoSignal : {COUNT3=0,ID3_message_ALTU=0,C=0,STOP=0}
    VINP_FAT_flg1 -> (junction 97) [order 1] : [VINP_TPMSResButt_flg||COUNT3==40||BackFlg==1]
    VINP_FAT_flg0 -> (junction 105) [order 1] : [VINP_TPMSResButt_flg||BackFlg==1]
    VINP_FAT_flg1 -> fivesec [order 2] : [after(500,tick)]
    VINP_FAT_flg0 -> fivesec [order 2] : [after(500,tick)]
  state time_cal [parallel]
    settings: executionOrder=2
    state cal1
      en:
      time_cal=time_cal+1
    state default
      en:
      time_cal=0
      BackFlg=0
    state back
      en:
      BackFlg=1
    (default) -> default
    default -> cal1 : [after(6400,tick)]{BackFlg=0}
    back -> default
    cal1 -> back [order 1] : [VINP_TPMSResButt_flg||time_cal>9]
    cal1 -> cal1 [order 2] : [after(6400,tick)]
  data: VINP_IDin_raw32 input; VINP_TPMSResButt_flg input; VINP_DATAin_flg input; S3IDLock input; COUNT3 output uint8; VINP_FAT_flg input; IDout input; ID3_message_ALTU output uint8; STOP local boolean; C local uint8; BackFlg local boolean; time_cal local uint8

== stateflow chart tpm/TPM/TPMS/TPMS/Learn/AutoLocation/IDIdentify/Acceptancerate/Chart5 ==
  state SensorReceived [parallel]
    settings: executionOrder=1
    state VINP_TPMSResButt_flg
      en:
      COUNT4=0;
      ID4_message_ALTU=0;
      C=0;
      STOP=0;
      BackFlg=0;
    state NoSignal
    state VINP_FAT_flg1
      en:
      COUNT4=COUNT4 +1
      C=0
    state VINP_FAT_flg0
      en:
      C=C+1
      ID4_message_ALTU=ID4_message_ALTU+1
    state fivesec
    (default) -> VINP_TPMSResButt_flg
    VINP_TPMSResButt_flg -> NoSignal
    NoSignal -> VINP_TPMSResButt_flg [order 1] : [VINP_TPMSResButt_flg||BackFlg==1]
    NoSignal -> (junction 57) [order 2] : [VINP_DATAin_flg&VINP_IDin_raw32==IDout&S4IDLock&VINP_FAT_flg==1&STOP==0]
    NoSignal -> (junction 61) [order 3] : [VINP_DATAin_flg&VINP_IDin_raw32==IDout&S4IDLock&VINP_FAT_flg==0]
    (junction 57) -> VINP_FAT_flg1
    (junction 61) -> VINP_FAT_flg0
    (junction 97) -> NoSignal : {COUNT4=0,ID4_message_ALTU=0,C=0,STOP=0}
    fivesec -> NoSignal [order 2]
    fivesec -> NoSignal [order 1] : [C==5]{STOP=1;C=0;}
    (junction 105) -> NoSignal : {COUNT4=0,ID4_message_ALTU=0,C=0,STOP=0}
    VINP_FAT_flg1 -> (junction 97) [order 1] : [VINP_TPMSResButt_flg||COUNT4==40||BackFlg==1]
    VINP_FAT_flg0 -> (junction 105) [order 1] : [VINP_TPMSResButt_flg||BackFlg==1]
    VINP_FAT_flg1 -> fivesec [order 2] : [after(500,tick)]
    VINP_FAT_flg0 -> fivesec [order 2] : [after(500,tick)]
  state time_cal [parallel]
    settings: executionOrder=2
    state cal1
      en:
      time_cal=time_cal+1
    state default
      en:
      time_cal=0
      BackFlg=0
    state back
      en:
      BackFlg=1
    (default) -> default
    default -> cal1 : [after(6400,tick)]{BackFlg=0}
    back -> default
    cal1 -> back [order 1] : [VINP_TPMSResButt_flg||time_cal>9]
    cal1 -> cal1 [order 2] : [after(6400,tick)]
  data: VINP_IDin_raw32 input; VINP_TPMSResButt_flg input; VINP_DATAin_flg input; S4IDLock input; COUNT4 output uint8; VINP_FAT_flg input; IDout input; ID4_message_ALTU output uint8; STOP local boolean; C local uint8; BackFlg local boolean; time_cal local uint8

== matlab function tpm/TPM/TPMS/TPMS/Learn/LowerTirePressureCalibration/PalarmSwitch ==
  data: LFP output; P1 input; P2 input; P3 input; P4 input; S1L input; S2L input; S3L input; S4L input; RFP output; LRP output; RRP output
function [LFP,RFP,LRP,RRP] = fcn(P1,P2,P3,P4,S1L,S2L,S3L,S4L)
P=[P1 P2 P3 P4];
S=[S1L S2L S3L S4L];
LFP=uint8(0);
RFP=uint8(0);
LRP=uint8(0);
RRP=uint8(0);
for i=1:length(S)
    if S(i)==1
        LFP=uint8(P(i));
    elseif S(i)==2
        RFP=uint8(P(i));
    elseif S(i)==3
        LRP=uint8(P(i));
    elseif S(i)==4
        RRP=uint8(P(i));
    end
end

== stateflow chart tpm/TPM/TPMS/TPMS/Learn/LowerTirePressureCalibration/Chart ==
  state LEFTFRONT [parallel]
    settings: executionOrder=1
    state FLASH
      en:
      VTPM_P1alarm_raw=VINP_FlashLFWheelPSW_raw8;
      VTPM_P1Pressindi_enum=VINP_FlashLFPindi_enum;
    state Autolocationpsw
      (default) -> (junction 228)
      LEFTFRONT.Autolocationpsw -> (junction 228) [order 1]
      (junction 228) -> (junction 222) [order 1] : [VTPM_S1pressindi_enum==1||VTPM_S1pressindi_enum==2]
      (junction 228) -> (junction 223) [order 2] : {VTPM_P1Pressindi_enum=VTPM_S1pressindi_enum;}
      (junction 222) -> (junction 224) : {VTPM_P1alarm_raw=VTPM_S1Palarm_raw;
          | VTPM_P1Pressindi_enum=VTPM_S1pressindi_enum;}
      (junction 224) -> (junction 223)
    state CaliandReset
      en:
      VTPM_P1alarm_raw=93;
      VTPM_P1Pressindi_enum=0;
    state Manualpsw
      en:
      VTPM_P1alarm_raw=VTPM_ManualP1alarm_raw;
      VTPM_P1Pressindi_enum=VTPM_ManuS1pressindi_enum;
    (default) -> (junction 260)
    (junction 260) -> LEFTFRONT.FLASH [order 1] : [VTPM_LocationDone_flg&&VINP_FlashLFPindi_enum != 0 && VINP_FlashLFPindi_enum != 3]
    (junction 260) -> LEFTFRONT.Autolocationpsw [order 2]
    LEFTFRONT.FLASH -> LEFTFRONT.CaliandReset : [VINP_TPMSResButt_flg||VINP_TPMSCaliButt_flg]
    LEFTFRONT.CaliandReset -> LEFTFRONT.Autolocationpsw
    LEFTFRONT.Manualpsw -> LEFTFRONT.CaliandReset [order 1] : [VINP_TPMSResButt_flg||VINP_TPMSCaliButt_flg]
    LEFTFRONT.Autolocationpsw -> LEFTFRONT.CaliandReset [order 1] : [VINP_TPMSResButt_flg||VINP_TPMSCaliButt_flg]
    LEFTFRONT.Autolocationpsw -> LEFTFRONT.Manualpsw [order 2] : [VTPM_TPMSmanualDone_flg]
    LEFTFRONT.Manualpsw -> LEFTFRONT.Manualpsw [order 2] : [VTPM_TPMSmanualDone_flg]
  state REARFORNT [parallel]
    settings: executionOrder=2
    state FLASH
      en:
      VTPM_P2alarm_raw=VINP_FlashRFWheelPSW_raw8;
      VTPM_P2Pressindi_enum=VINP_FlashRFPindi_enum;
    state Autolocationpsw
      (default) -> (junction 310)
      REARFORNT.Autolocationpsw -> (junction 310) [order 1]
      (junction 310) -> (junction 325) [order 1] : [VTPM_S2pressindi_enum==1||VTPM_S2pressindi_enum==2]
      (junction 310) -> (junction 309) [order 2] : {VTPM_P2Pressindi_enum=VTPM_S2pressindi_enum;}
      (junction 325) -> (junction 308) : {VTPM_P2alarm_raw=VTPM_S2Palarm_raw;
          | VTPM_P2Pressindi_enum=VTPM_S2pressindi_enum;}
      (junction 308) -> (junction 309)
    state CaliandReset
      en:
      VTPM_P2alarm_raw=93;
      VTPM_P2Pressindi_enum=0;
    state Manualpsw
      en:
      VTPM_P2alarm_raw=VTPM_ManualP2alarm_raw;
      VTPM_P2Pressindi_enum=VTPM_ManuS2pressindi_enum;
    (default) -> (junction 317)
    (junction 317) -> REARFORNT.FLASH [order 1] : [VTPM_LocationDone_flg&&VINP_FlashRFPindi_enum != 0 && VINP_FlashRFPindi_enum != 3]
    (junction 317) -> REARFORNT.Autolocationpsw [order 2]
    REARFORNT.FLASH -> REARFORNT.CaliandReset : [VINP_TPMSResButt_flg||VINP_TPMSCaliButt_flg]
    REARFORNT.CaliandReset -> REARFORNT.Autolocationpsw
    REARFORNT.Manualpsw -> REARFORNT.CaliandReset [order 1] : [VINP_TPMSResButt_flg||VINP_TPMSCaliButt_flg]
    REARFORNT.Autolocationpsw -> REARFORNT.CaliandReset [order 1] : [VINP_TPMSResButt_flg||VINP_TPMSCaliButt_flg]
    REARFORNT.Autolocationpsw -> REARFORNT.Manualpsw [order 2] : [VTPM_TPMSmanualDone_flg]
    REARFORNT.Manualpsw -> REARFORNT.Manualpsw [order 2] : [VTPM_TPMSmanualDone_flg]
  state LEFTREAR [parallel]
    settings: executionOrder=3
    state FLASH
      en:
      VTPM_P3alarm_raw=VINP_FlashLRWheelPSW_raw8;
      VTPM_P3Pressindi_enum=VINP_FlashLRPindi_enum;
    state Autolocationpsw
      (default) -> (junction 334)
      LEFTREAR.Autolocationpsw -> (junction 334) [order 1]
      (junction 334) -> (junction 349) [order 1] : [VTPM_S3pressindi_enum==1||VTPM_S3pressindi_enum==2]
      (junction 334) -> (junction 335) [order 2] : {VTPM_P3Pressindi_enum=VTPM_S3pressindi_enum;}
      (junction 349) -> (junction 333) : {VTPM_P3alarm_raw=VTPM_S3Palarm_raw;
          | VTPM_P3Pressindi_enum=VTPM_S3pressindi_enum;}
      (junction 333) -> (junction 335)
    state CaliandReset
      en:
      VTPM_P3alarm_raw=93;
      VTPM_P3Pressindi_enum=0;
    state Manualpsw
      en:
      VTPM_P3alarm_raw=VTPM_ManualP3alarm_raw;
      VTPM_P3Pressindi_enum=VTPM_ManuS3pressindi_enum;
    (default) -> (junction 332)
    (junction 332) -> LEFTREAR.FLASH [order 1] : [VTPM_LocationDone_flg&&VINP_FlashLRPindi_enum != 0 && VINP_FlashLRPindi_enum != 3]
    (junction 332) -> LEFTREAR.Autolocationpsw [order 2]
    LEFTREAR.FLASH -> LEFTREAR.CaliandReset : [VINP_TPMSResButt_flg||VINP_TPMSCaliButt_flg]
    LEFTREAR.CaliandReset -> LEFTREAR.Autolocationpsw
    LEFTREAR.Manualpsw -> LEFTREAR.CaliandReset [order 1] : [VINP_TPMSResButt_flg||VINP_TPMSCaliButt_flg]
    LEFTREAR.Autolocationpsw -> LEFTREAR.CaliandReset [order 1] : [VINP_TPMSResButt_flg||VINP_TPMSCaliButt_flg]
    LEFTREAR.Autolocationpsw -> LEFTREAR.Manualpsw [order 2] : [VTPM_TPMSmanualDone_flg]
    LEFTREAR.Manualpsw -> LEFTREAR.Manualpsw [order 2] : [VTPM_TPMSmanualDone_flg]
  state RIGHTREAR [parallel]
    settings: executionOrder=4
    state FLASH
      en:
      VTPM_P4alarm_raw=VINP_FlashRRWheelPSW_raw8;
      VTPM_P4Pressindi_enum=VINP_FlashRRPindi_enum;
    state Autolocationpsw
      (default) -> (junction 357)
      RIGHTREAR.Autolocationpsw -> (junction 357) [order 1]
      (junction 357) -> (junction 372) [order 1] : [VTPM_S4pressindi_enum==1||VTPM_S4pressindi_enum==2]
      (junction 357) -> (junction 358) [order 2] : {VTPM_P4Pressindi_enum=VTPM_S4pressindi_enum;}
      (junction 372) -> (junction 356) : {VTPM_P4alarm_raw=VTPM_S4Palarm_raw;
          | VTPM_P4Pressindi_enum=VTPM_S4pressindi_enum;}
      (junction 356) -> (junction 358)
    state CaliandReset
      en:
      VTPM_P4alarm_raw=93;
      VTPM_P4Pressindi_enum=0;
    state Manualpsw
      en:
      VTPM_P4alarm_raw=VTPM_ManualP4alarm_raw;
      VTPM_P4Pressindi_enum=VTPM_ManuS4pressindi_enum;
    (default) -> (junction 355)
    (junction 355) -> RIGHTREAR.FLASH [order 1] : [VTPM_LocationDone_flg&&VINP_FlashRRPindi_enum != 0 && VINP_FlashRRPindi_enum != 3]
    (junction 355) -> RIGHTREAR.Autolocationpsw [order 2]
    RIGHTREAR.FLASH -> RIGHTREAR.CaliandReset : [VINP_TPMSResButt_flg||VINP_TPMSCaliButt_flg]
    RIGHTREAR.CaliandReset -> RIGHTREAR.Autolocationpsw
    RIGHTREAR.Manualpsw -> RIGHTREAR.CaliandReset [order 1] : [VINP_TPMSResButt_flg||VINP_TPMSCaliButt_flg]
    RIGHTREAR.Autolocationpsw -> RIGHTREAR.CaliandReset [order 1] : [VINP_TPMSResButt_flg||VINP_TPMSCaliButt_flg]
    RIGHTREAR.Autolocationpsw -> RIGHTREAR.Manualpsw [order 2] : [VTPM_TPMSmanualDone_flg]
    RIGHTREAR.Manualpsw -> RIGHTREAR.Manualpsw [order 2] : [VTPM_TPMSmanualDone_flg]
  data: VINP_FlashLFPindi_enum input; VINP_FlashLFWheelPSW_raw8 input; VINP_FlashLRPindi_enum input; VINP_FlashLRWheelPSW_raw8 input; VINP_FlashRFPindi_enum input; VINP_FlashRFWheelPSW_raw8 input; VINP_FlashRRPindi_enum input; VINP_FlashRRWheelPSW_raw8 input; VTPM_S1Palarm_raw input; VTPM_S1pressindi_enum input; VTPM_S2Palarm_raw input; VTPM_S2pressindi_enum input; VTPM_S3Palarm_raw input; VTPM_S3pressindi_enum input; VTPM_S4Palarm_raw input; VTPM_S4pressindi_enum input; VTPM_P1alarm_raw output uint8; VTPM_P2alarm_raw output uint8; VTPM_P3alarm_raw output uint8; VTPM_P4alarm_raw output uint8; VTPM_P1Pressindi_enum output uint8; VTPM_P2Pressindi_enum output uint8; VTPM_P3Pressindi_enum output uint8; VTPM_P4Pressindi_enum output uint8; VTPM_TPMSmanualDone_flg input; VTPM_ManuS1pressindi_enum input; VTPM_ManuS2pressindi_enum input; VTPM_ManuS3pressindi_enum input; VTPM_ManuS4pressindi_enum input; VTPM_ManualP1alarm_raw input; VTPM_ManualP2alarm_raw input; VTPM_ManualP3alarm_raw input; VTPM_ManualP4alarm_raw input; VINP_TPMSCaliButt_flg input; VINP_TPMSResButt_flg input; VTPM_LocationDone_flg input

== stateflow chart tpm/TPM/TPMS/TPMS/Send/DATA/LFSW ==
  state OFF
  state ON
    state Reset_Cail
      en:
      VTPM_LFWheelTemp_C=215;
    state StandBy
    state Received
      en:VTPM_LFWheelPress_raw8=VINP_Pin_raw8;
      VTPM_LFWheelTemp_C=VTPM_Tin_c;
      VTPM_LFBatWarn_flg=VINP_BatteryLow_flg;
      VTPM_LFP20_raw8=uint8(((double(VTPM_LFWheelPress_raw8)*1.72+151)*(273+20)/(273+double(VTPM_LFWheelTemp_C))-151)/1.72);
      VTPM_LFWheelDebug_flg=true;
      VTPM_LFSensorMode_flg=VINP_FAT_flg;
      VTPM_LFSensorFail_flg=false;
      ex:
      VTPM_LFWheelDebug_flg=false;
      VTPM_LFSensorMode_flg=false;
    state PreSenfail
    state SensorFail
      en:VTPM_LFSensorFail_flg=true;
    (default) -> StandBy
    StandBy -> Reset_Cail [order 1] : [VINP_TPMSResButt_flg]
    Reset_Cail -> StandBy
    StandBy -> Received [order 2] : [VTPM_LFSW_flg==true]
    Received -> StandBy : [VTPM_LFSW_flg==false]
    SensorFail -> StandBy [order 2] : [!VTPM_Done_flg]
        | {VTPM_LFSensorFail_flg=false;
        | }
    PreSenfail -> StandBy [order 2] : [VINP_VehSpeed_kph<25||!VTPM_Done_flg]
    StandBy -> PreSenfail [order 3] : [VINP_VehSpeed_kph>=25&&VTPM_Done_flg]
    PreSenfail -> Received [order 1] : [VTPM_LFSW_flg==true]
    SensorFail -> Received [order 1] : [VTPM_LFSW_flg==true]
    PreSenfail -> SensorFail [order 3] : [after(48000,tick)]
  (default) -> OFF
  ON -> OFF : [VPMM_PowerSta_enum==ENUM_POWERSTA_OFF||...
      | VPMM_PowerSta_enum==ENUM_POWERSTA_OFFC||...
      | VPMM_PowerSta_enum==ENUM_POWERSTA_OFFA||...
      | VPMM_PowerSta_enum==ENUM_POWERSTA_STANDBY
      | ]
  OFF -> ON : [VPMM_PowerSta_enum==ENUM_POWERSTA_ON||...
      | VPMM_PowerSta_enum==ENUM_POWERSTA_READY]
  data: VTPM_LFSW_flg input; VINP_Pin_raw8 input; VTPM_Tin_c input; VINP_BatteryLow_flg input; VTPM_LFWheelPress_raw8 output uint8; VTPM_LFWheelTemp_C output single; VTPM_LFBatWarn_flg output boolean; VTPM_LFSensorFail_flg output boolean; VPMM_PowerSta_enum input; VTPM_LFP20_raw8 output uint8; VINP_FAT_flg input; VTPM_LFWheelDebug_flg output boolean; VTPM_LFSensorMode_flg output boolean; ENUM_POWERSTA_ON parameter; ENUM_POWERSTA_READY parameter; VINP_VehSpeed_kph input; VTPM_Done_flg input; ENUM_POWERSTA_OFF parameter; ENUM_POWERSTA_OFFA parameter; ENUM_POWERSTA_OFFC parameter; ENUM_POWERSTA_STANDBY parameter; VINP_TPMSResButt_flg input

== stateflow chart tpm/TPM/TPMS/TPMS/Learn/AutoLocation/WheelPosition/Chart5 ==
  state Start
    state Forward
      en:
      a=(VTPM_RRWpos_raw+Delta);
      b=(VTPM_RRWpos_raw+Delta)/96;
      VTPM_RRWpos_raw=a-b*96;
    state Else
    state Backward
      en:
      a=(VTPM_RRWpos_raw+Delta);
      b=(VTPM_RRWpos_raw+Delta)/96;
      VTPM_RRWpos_raw=a-b*96;
    (default) -> (junction 54) : {VTPM_RRWpos_raw=0; Delta=0; PulseCountBuf=VINP_RRPulseCount_cnt;}
    Start -> (junction 54) : [hasChanged(VINP_RRPulseCount_cnt)]....
        | {Delta=VINP_RRPulseCount_cnt-PulseCountBuf;
        | PulseCountBuf=VINP_RRPulseCount_cnt;}
    (junction 54) -> (junction 47) [order 1] : [VPMM_PowerSta_enum!=ENUM_PWRSTASW_OFF&&....
        |  VPMM_PowerSta_enum!=ENUM_PWRSTASW_OFFCHVCHRG&&...
        |  VPMM_PowerSta_enum!=ENUM_PWRSTASW_OFFA&&....
        |  VPMM_PowerSta_enum!=ENUM_PWRSTASW_STANDBY&&....
        |  VINP_RRPulseCountV_flg==false]
    (junction 47) -> (junction 6) [order 1] : [VTPM_RRWhlRotDir_enum==1]
    (junction 6) -> Forward [order 1] : [Delta>0]
    (junction 54) -> Else [order 2]
    (junction 47) -> (junction 48) [order 2]
    (junction 6) -> (junction 10) [order 2] : [Delta<0]
    (junction 10) -> Forward : {Delta=Delta+256;}
    (junction 48) -> Else [order 2]
    (junction 48) -> (junction 14) [order 1] : [VTPM_RRWhlRotDir_enum==2]
    (junction 14) -> Backward [order 1] : [Delta>0]{Delta=-Delta+96;}
    (junction 14) -> (junction 16) [order 2] : [Delta<0]
    (junction 16) -> Backward : {Delta=-Delta+128;}
  data: VPMM_PowerSta_enum input; VINP_RRPulseCount_cnt input; VINP_RRPulseCountV_flg input; VTPM_RRWhlRotDir_enum input; VTPM_RRWpos_raw output int16; a local int16; b local int16; Delta local int16; PulseCountBuf local int16; ENUM_PWRSTASW_OFF parameter; ENUM_PWRSTASW_OFFA parameter; ENUM_PWRSTASW_OFFCHVCHRG parameter; ENUM_PWRSTASW_STANDBY parameter
